simulink model "DC_motor_PIDAW_d"  (R2015b)
settings: Solver=VariableStepAuto  StartTime=0.0  StopTime=10  MaxStep=1e-2  RelTol=1e-3
settings Model: Creator=mgreiff  LastModifiedBy=mgreiff
settings DebuggingCC: AlgebraicLoopMsg=none

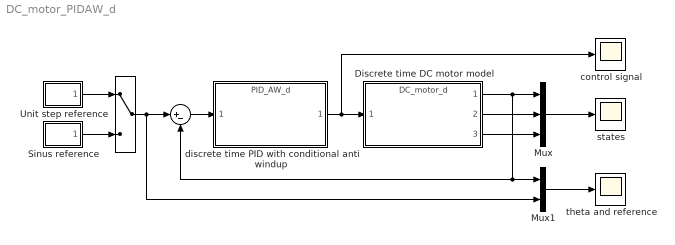
== system DC_motor_PIDAW_d ==
  " " : Sum  Inputs=|+-
  "   " : ManualSwitch
  Discrete time DC motor model : ModelReference  ModelNameDialog=DC_motor_d.slx  SimulationMode=Normal  ModelReferenceVersion=1.8  CopyOfModelName=DC_motor_d.slx
  Mux : Mux  Inputs=3
  Mux1 : Mux  Inputs=2
  Sinus reference : Subsystem
  Unit step reference : Subsystem
  control signal : Scope
  discrete time PID with conditional anti windup : ModelReference  ModelNameDialog=PID_AW_d.slx  SimulationMode=Normal  ModelReferenceVersion=1.8  CopyOfModelName=PID_AW_d.slx
  states : Scope
  theta and reference : Scope
  wires:
  Discrete time DC motor model/1 -> " "/2, Mux1/1, Mux/1
  Discrete time DC motor model/2 -> Mux/2
  Discrete time DC motor model/3 -> Mux/3
  Mux/1 -> states/1
  Unit step reference/1(voltage) -> "   "/1
  Sinus reference/1(voltage) -> "   "/2
  discrete time PID with conditional anti windup/1 -> control signal/1, Discrete time DC motor model/1
  "   "/1 -> Mux1/2, " "/1
  " "/1 -> discrete time PID with conditional anti windup/1
  Mux1/1 -> theta and reference/1

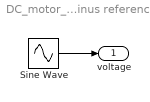
== system DC_motor_PIDAW_d/Sinus reference ==
  Sine Wave : Sin  Frequency=2*pi/10  SampleTime=0
  voltage : Outport
  wires:
  Sine Wave/1 -> voltage/1

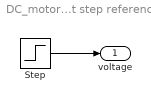
== system DC_motor_PIDAW_d/Unit step reference ==
  Step : Step  Time=0  SampleTime=0
  voltage : Outport
  wires:
  Step/1 -> voltage/1
